simulink model "Control_test"  (R2014b)
settings: Solver=FixedStepDiscrete  StartTime=0.0  StopTime=Inf  FixedStep=0.001  RelTol=1e-3
PostLoadFcn:
  | , if any(exist('dsrtsu_mdlpostloadfcn', 'file') == [2, 3, 6]), try dsrtsu_mdlpostloadfcn('Execute', bdroot); catch fprintf('Error in PostLoadFcn (dsrtsu_mdlpostloadfcn) for model "%s":\n %s\n', bdroot, lasterr); end, end,
undefined symbols (not defined in the file or in its folder): dtLocal, slcm
libraries: rtican x163, simulink x14
(part 34 of 34)

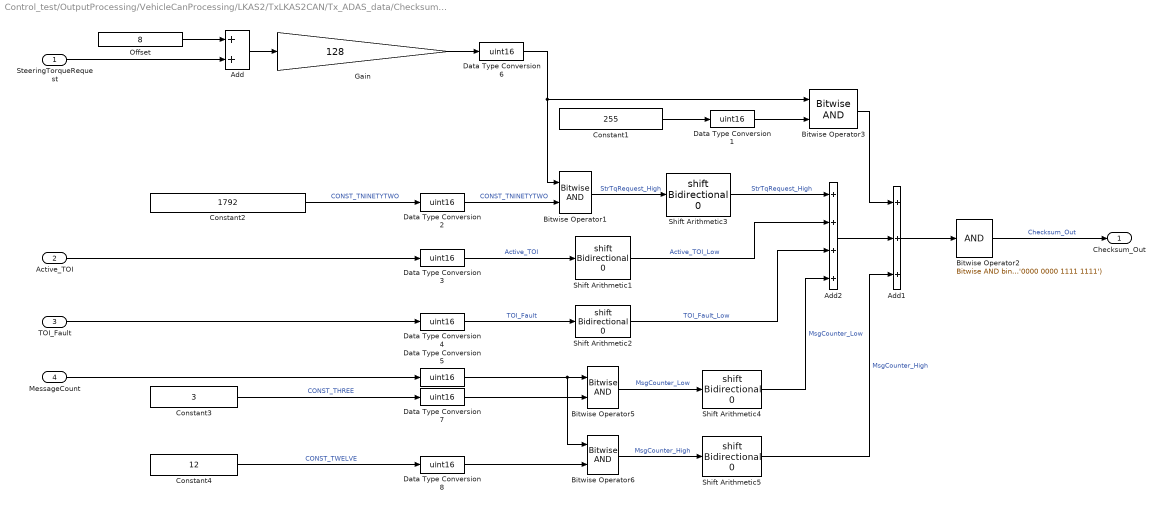
== system Control_test/OutputProcessing/VehicleCanProcessing/LKAS2/TxLKAS2CAN/Tx_ADAS_data/Checksum_NEW ==
  SteeringTorqueRequest : Inport
  Active_TOI : Inport  Port=2
  TOI_Fault : Inport  Port=3
  MessageCount : Inport  Port=4
  Add : Sum
  Add1 : Sum  Inputs=+++  OutDataTypeStr=uint16
  Add2 : Sum  Inputs=++++  OutDataTypeStr=uint16
  Bitwise Operator{1,3,5..6} (4 alike) : simulink/Logic and Bit Operations/Bitwise Operator  logicop=AND  UseBitMask=off  NumInputPorts=2  BitMask=bin2dec('0000 0000 1111 1111')  BitMaskRealWorld=Stored Integer
  Bitwise Operator2 : simulink/Logic and Bit Operations/Bitwise Operator  logicop=AND  UseBitMask=on  BitMask=bin2dec('0000 0000 1111 1111')  BitMaskRealWorld=Stored Integer
  Constant1 : Constant  Value=255
  Constant2 : Constant  Value=1792
  Constant3 : Constant  Value=3
  Constant4 : Constant  Value=12
  Data Type Conversion{1..8} (8 alike) : DataTypeConversion  OutDataTypeStr=uint16
  Gain : Gain  Gain=128
  Offset : Constant  Value=8
  Shift Arithmetic{1..5} (5 alike) : ArithShift
  Checksum_Out : Outport
  wires:
  SteeringTorqueRequest/1 -> Add/2
  Gain/1 -> Data Type Conversion6/1
  Offset/1 -> Add/1
  Add/1 -> Gain/1
  Bitwise Operator2/1 -> Checksum_Out/1  "Checksum_Out"
  MessageCount/1 -> Data Type Conversion5/1
  TOI_Fault/1 -> Data Type Conversion4/1
  Active_TOI/1 -> Data Type Conversion3/1
  Add2/1 -> Add1/2
  Shift Arithmetic2/1 -> Add2/3  "TOI_Fault_Low"
  Shift Arithmetic4/1 -> Add2/4  "MsgCounter_Low"
  Shift Arithmetic5/1 -> Add1/3  "MsgCounter_High"
  Bitwise Operator6/1 -> Shift Arithmetic5/1  "MsgCounter_High"
  Data Type Conversion8/1 -> Bitwise Operator6/2
  Constant4/1 -> Data Type Conversion8/1  "CONST_TWELVE"
  Bitwise Operator5/1 -> Shift Arithmetic4/1  "MsgCounter_Low"
  Data Type Conversion7/1 -> Bitwise Operator5/2
  Constant3/1 -> Data Type Conversion7/1  "CONST_THREE"
  Data Type Conversion5/1 -> Bitwise Operator6/1, Bitwise Operator5/1
  Data Type Conversion4/1 -> Shift Arithmetic2/1  "TOI_Fault"
  Shift Arithmetic1/1 -> Add2/2  "Active_TOI_Low"
  Data Type Conversion3/1 -> Shift Arithmetic1/1  "Active_TOI"
  Shift Arithmetic3/1 -> Add2/1  "StrTqRequest_High"
  Bitwise Operator3/1 -> Add1/1
  Bitwise Operator1/1 -> Shift Arithmetic3/1  "StrTqRequest_High"
  Data Type Conversion2/1 -> Bitwise Operator1/2  "CONST_TNINETYTWO"
  Constant2/1 -> Data Type Conversion2/1  "CONST_TNINETYTWO"
  Data Type Conversion1/1 -> Bitwise Operator3/2
  Constant1/1 -> Data Type Conversion1/1
  Data Type Conversion6/1 -> Bitwise Operator1/1, Bitwise Operator3/1
  Add1/1 -> Bitwise Operator2/1

== system Control_test/OutputProcessing/VehicleCanProcessing/LKAS2/TxLKAS2CAN/MessageCounter/Shinho Systems Co., Ltd./Model Info ==
  EmptySubsystem : Subsystem

== system Control_test/OutputProcessing/VehicleCanProcessing/LKAS2/TxLKAS2CAN/MessageCounter/Shinho Systems Co., Ltd./Model Info/EmptySubsystem ==

== matlab function Control_test/Controller/CalBelief Subsystem/MATLAB Function1 ==
  data: b_q input; b_q_next output; xk input; x_next input; sigma input; b_x_next output; reactiveDist input; safeDist input
function [b_q_next, b_x_next] = CalBelief(b_q, xk, x_next, sigma, reactiveDist, safeDist)

nDState = length(b_q);
b_q_next = zeros(nDState, 1);

if (norm(x_next - xk) < 1e-6)
    b_q_next = b_q;
else
    
    for qq = 1:nDState
        tmp = 0;
        for q = 1:nDState
            tmp = tmp + DStateTransfn(qq, q, sigma) * b_q(q);
        end
        b_q_next(qq) = DObsfn(0, qq) * ...
                       CStateTransfn(x_next, qq, xk, reactiveDist, safeDist) * tmp;
    end

    if (sum(b_q_next) == 0)
        b_q_next = b_q;
    else
        b_q_next = b_q_next / sum(b_q_next);
    end
end

b_x_next = x_next;

end

== matlab function Control_test/Controller/MATLAB Function ==
  data: x_in input; d_out output; y_in input; theta_in input; v_in input; x_ori input; y_ori input; theta_ori input; v_out output
function [d_out, v_out] = Global2Local(x_in, y_in, theta_in, v_in, x_ori, y_ori, theta_ori)

temp = [cos(-theta_ori) -sin(theta_ori);...
       sin(theta_ori) cos(theta_ori)] * [x_in - x_ori; y_in - y_ori];
x_local = temp(1);
theta_local = theta_in - theta_ori;

d_out = x_local;
v_out = v_in * cos(theta_local);

end

== matlab function Control_test/Controller/MATLAB Function2 ==
  data: b_q input; control_discrete output; x input; nAlphas input; sigmas input; localxs input; params input; safeDist input; u output
function [control_discrete, u] = FindOptimalContol(b_q, x, nAlphas, sigmas, localxs, params, safeDist)

nCState = length(x);
localxs = reshape(localxs, nCState, []);
params = reshape(params, 21, 12, []);
thresholddist = 10;
nDState = length(b_q);

bestvalue = -1e20;
bestidx = -1;

mindist = 1e20;
mindistidx = -1;

for n = 1:nAlphas
    sum  = 0;
    dist = norm(x - localxs(:, n));
    if (dist < thresholddist && (SatisfyConstraints(x, safeDist) || ...
		                         ~SatisfyConstraints(localxs(:, n), safeDist)))
        for q = 1:nDState
            const_term = params(1, q, n);
            first_order_term = params(2:(1+nCState), q, n);
            second_order_term = params((2+nCState):(1+nCState+nCState*nCState), q, n);
            second_order_term_reshape = reshape(second_order_term, nCState, nCState);
            sum = sum + b_q(q) * (const_term + first_order_term' * (x - localxs(:, n)) + ...
                                  (x - localxs(:, n))' * second_order_term_reshape * (x - localxs(:, n)));
        end
        
        if (sum > bestvalue)
            bestvalue = sum;
            bestidx = n;
        end
    end
    if (dist < mindist)
        mindist = dist;
        mindistidx = n;
    end
end

if (bestidx == -1)
    bestidx = mindistidx;
    disp('No point within the threshold, use policy with the nearest point.');
end

control_discrete = sigmas(bestidx);
disp('control_discrete = ');
disp(control_discrete);

if (control_discrete == 1) 
    u = 0;
elseif (control_discrete == 2)
    u = 1;
else
    u = -1;
end


end

== matlab function Control_test/Controller/MATLAB Function4 ==
  data: q_h_next input; x_h output; x_k input; reactionDist input; v_h output; safeDist input
function [x_h, v_h] = HumanDriverStateSimulator(q_h_next, x_k, reactionDist, safeDist)

if (~SatisfyConstraints(x_k, safeDist))
    x_h =  x_k(1);
    v_h =  x_k(2);
    
else
    OBLIVIOUS = 1; AGGRESSIVE = 2; COURTEOUS = 3; REASONABLE = 4;
    mNoiseMean = 0;
    mDistNoiseStd = 0.1;
    mVelNoiseStd = 0.1;
    mDeltaT = 0.1;

    humanDriver = q_h_next;

    if (humanDriver == OBLIVIOUS)
            humanInput = 0;
    elseif (humanDriver == AGGRESSIVE)
        if (abs(x_k(1) - x_k(3)) < reactionDist)
            humanInput = 1;
        else
            humanInput = 0;
        end
    elseif (humanDriver == COURTEOUS)
        if (abs(x_k(1) - x_k(3)) < reactionDist)
            humanInput = -1; 
        else
            humanInput = 0;
        end
    elseif (humanDriver == REASONABLE)
        if (abs(x_k(1) - x_k(3)) < reactionDist)
            if (x_k(2) > x_k(4))
                humanInput = 1;
            else
                humanInput = -1;
            end
        else
            humanInput = 0;
        end
    else
        humanInput = 0;
        disp('SampleHumanDriverState: q_next out of domain');
    end
    
    distNoise4HumanDriver = normrnd(mNoiseMean, mDistNoiseStd);
    velNoise4HumanDriver = normrnd(mNoiseMean, mVelNoiseStd);
    
    x_h = x_k(1) + mDeltaT * x_k(2) + distNoise4HumanDriver;
    v_h = x_k(2) + mDeltaT * humanInput + velNoise4HumanDriver;
end


end

== matlab function Control_test/InputProcessing/CameraCanProcessing/CameraPT ==
  data: u input; TargetDist output; TargetRelSpeed output
function [TargetDist, TargetRelSpeed] = CameraObjProcessing(u)
%#codegen

% Inputs
CIPV = u(1:8);
Range = u(9:16);
RangeRate = u(17:24);

% Outputs
TargetDist = CIPV'*Range;
TargetRelSpeed = CIPV'*RangeRate;
% if TargetDist < 0.1
%     TargetDist = 170;
%     TargetRelSpeed = 30 - speed_ego;
% end

== matlab function Control_test/Controller/MATLAB Function3 ==
  data: x_in input; d_out output; y_in input; theta_in input; v_in input; x_ori input; y_ori input; theta_ori input; v_out output
function [d_out, v_out] = Global2Local(x_in, y_in, theta_in, v_in, x_ori, y_ori, theta_ori)


temp = [cos(-theta_ori) -sin(theta_ori);...
                      sin(theta_ori) cos(theta_ori)] * [x_in - x_ori; y_in - y_ori];
x_local = temp(1);
theta_local = theta_in - theta_ori;

d_out = x_local;
v_out = v_in * cos(theta_local);

end

== matlab function Control_test/SensorFusion/Map-based Localization/INS Reference Change ==
  data: PosLon input; PosLat input; GPS_Local_Pos output; AngleHeading input; Map2 parameter; INS_Heading output
function [GPS_Local_Pos,INS_Heading] = INSReferenceChange(PosLon,PosLat,AngleHeading,Map2)

[GPS_Local_Pos,INS_Heading] = INSReferenceChange(PosLon,PosLat,AngleHeading,Map2);

== matlab function Control_test/Controller/MATLAB Function1 ==
  data: x_r input; x_h output; y_r input; theta_r input; r input; theta input; y_h output; theta_h output
function [x_h, y_h, theta_h] = Sensor2EgoLocal(x_r, y_r, theta_r, r, theta)

theta_h = theta_r;
x_h = x_r +cos(theta);
y_h = y_r + sin(theta);

end

== matlab function Control_test/Controller/MATLAB Function5 ==
  data: q_h input; u input; q output
function q = Convert2DiscreteState(q_h, u)

if (u > 0)
    q_r  = 2;
elseif (u < 0)
    q_r = 3;
else
    q_r = 1;
end

q = (q_h - 1)*3 + q_r ;

end

== stateflow chart Control_test/OutputProcessing/TM_StateMachine ==
  state Communication
    state Abort
      du : T_Spas_Stat = 7;
    state Standby
      du : T_Spas_Stat = 3;
    state Control_ON
      du : T_Spas_Stat = 5;
    state Failure
      du : T_Spas_Stat = 6;
    (junction 24) -> Abort
    Abort -> (junction 32) : [T_SPAS_TM_CTRL_Mode == 0]
    Control_ON -> (junction 24) [order 2] : [TM_Stat == 7]
    (junction 32) -> Standby
    (junction 18) -> (junction 20) : [T_SPAS_TM_CTRL_Mode == 0]
    (junction 20) -> Standby
    Control_ON -> (junction 18) [order 1]
    Standby -> Control_ON [order 2] : [(TM_Stat == 5) &&...
        | (T_SPAS_TM_CTRL_Mode == 1)]
    Standby -> Failure [order 1] : [TM_Stat == 6]
    Control_ON -> (junction 26) [order 3] : [TM_Stat == 6]
    (junction 26) -> Failure
  state Init
    du : T_Spas_Stat = 1;
  state Interface_Start
    du : T_Spas_Stat = 2;
  (default) -> Init
  Init -> Interface_Start : [TM_Stat != 6]
  Communication -> Interface_Start : [TM_Stat == 2]
  Interface_Start -> Standby : [TM_Stat == 3]
  (junction 13) -> Interface_Start
  Failure -> (junction 13) : [TM_Stat == 6]
  data: T_SPAS_TM_CTRL_Mode input double; TM_Stat input double; T_Spas_Stat output double

== matlab function Control_test/Driver Override Logic/Driver Override Logic ==
  data: u input; y output; th_Tq input
function y = DriverOverrideLogic(u, th_Tq)
%#codegen

if ((round(u(1))~=0 && u(5)~=0) || u(6)==1 || (abs(u(7))>th_Tq && u(4)==1)) && (u(2)==1 || u(3)==1 || u(4)==1 || (u(5)>1 && u(5)<=4))
    y = 1;
else
    y = 0;
end
